simulink model "SecRwRtStFwdBkwdSpdCtrl"  (R2018b)
settings: Solver=FixedStepDiscrete  StartTime=0.0  StopTime=10.0  FixedStep=0.01  RelTol=1e-3
libraries: simulink x12
settings Model: Creator=sn2xws  LastModifiedBy=sn2xws
settings Model: ModifiedHistory=|
  | V2.4.0 Bug 655803  根据<REQ_MSM_697>修改调速
  | 2024.2.22
  | V2.5.0 Bug 732451增加模式15，18长滑轨调速
  | 2024.8.26 V3.0.0 557无长滑轨调速需求，发送默认值0
settings DataIOCC: SaveFormat=StructureWithTime
settings OptimizationCC: DefaultParameterBehavior=Inlined  EnhancedBackFolding=on  PassReuseOutputArgsAs=Individual arguments  ZeroExternalMemoryAtStartup=off  ZeroInternalMemoryAtStartup=off  OptimizeBlockOrder=speed  DifferentSizesBufferReuse=on  OptimizationCustomize=off
settings DebuggingCC: ParameterTunabilityLossMsg=error
settings ModelReferenceCC: ModelReferenceNumInstancesAllowed=Single
settings SFSimCC: MATLABDynamicMemAlloc=off
settings RTWCC: SystemTargetFile=autosar.tlc  GenCodeOnly=on  TemplateMakefile=ert_default_tmf  Description=AUTOSAR  GenerateReport=on  IncludeHyperlinkInReport=on  LaunchReport=on  GenerateTraceInfo=on  GenerateTraceReport=on  GenerateTraceReportSl=on  GenerateTraceReportSf=on  GenerateTraceReportEml=on  GenerateCodeMetricsReport=on
settings CodeAppCC: ForceParamTrailComments=on  IgnoreCustomStorageClasses=off  OperatorAnnotations=on  SimulinkDataObjDesc=on  SFDataObjDesc=on  InsertBlockDesc=on
settings STFCustomTargetCC: TargetLangStandard=C99 (ISO)  MultiwordLength=256  ParMdlRefBuildCompliant=on  CompOptLevelCompliant=on  IncludeMdlTerminateFcn=off  CombineOutputUpdateFcns=on  SuppressErrorStatus=on  ERTCustomFileBanners=on  SupportNonFinite=off  SupportComplex=off  SupportContinuousTime=off  SupportNonInlinedSFcns=off  RemoveResetFunc=on  MATLABClassNameForMDSCustomization=Simulink.SoftwareTarget.ERTCustomization  AutosarCompliant=on  UseToolchainInfoCompliant=on  LookupTableObjectStructAxisOrder=2,1,3,4,...  LUTObjectStructOrderEvenSpacing=Size,Table,Breakpoints  SystemTargetFile=autosar.tlc
settings ERTTargetCC: TargetLangStandard=C99 (ISO)  ConcurrentExecutionCompliant=off  IncludeMdlTerminateFcn=off  SuppressErrorStatus=on  SupportNonFinite=off  SupportComplex=off  ModelStepFunctionPrototypeControlCompliant=off  CPPClassGenCompliant=off  AutosarCompliant=on  LookupTableObjectStructAxisOrder=2,1,3,4,...  LUTObjectStructOrderEvenSpacing=Size,Table,Breakpoints  InlinedParameterPlacement=NonHierarchical  ERTCustomFileTemplate=example_file_process.tlc  ERTFilePackagingFormat=Compact

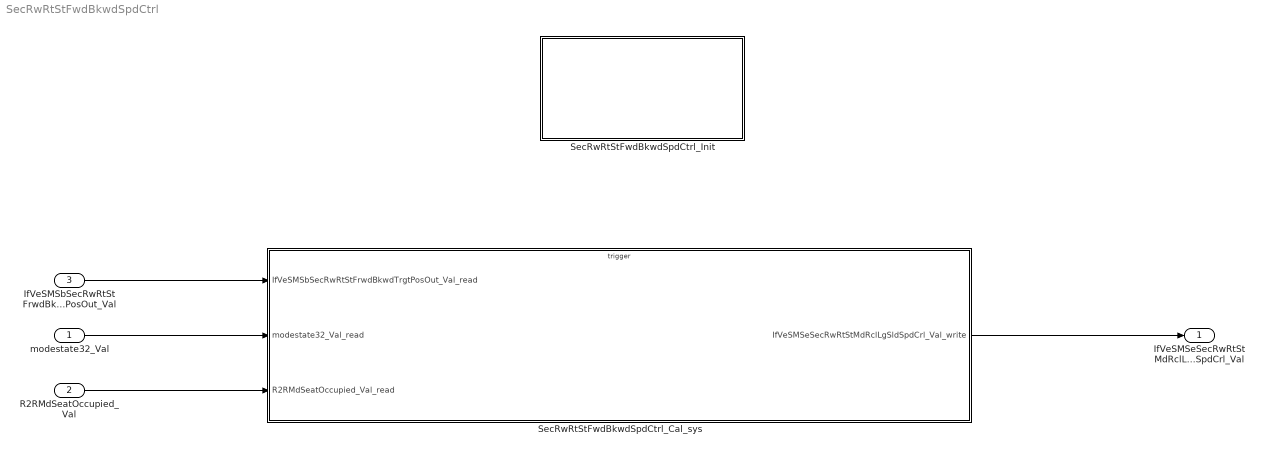
== system SecRwRtStFwdBkwdSpdCtrl ==
  modestate32_Val : Inport  OutDataTypeStr=uint32  PortDimensions=1
  R2RMdSeatOccupied_Val : Inport  Port=2  OutDataTypeStr=boolean  PortDimensions=1
  IfVeSMSbSecRwRtStFrwdBkwdTrgtPosOut_Val : Inport  Port=3  OutDataTypeStr=boolean  PortDimensions=1
  SecRwRtStFwdBkwdSpdCtrl_Cal_sys : Subsystem
  SecRwRtStFwdBkwdSpdCtrl_Init : Subsystem
  IfVeSMSeSecRwRtStMdRclLgSldSpdCrl_Val : Outport  OutDataTypeStr=uint8  PortDimensions=1
  wires:
  modestate32_Val/1 -> SecRwRtStFwdBkwdSpdCtrl_Cal_sys/2(modestate32_Val_read)
  R2RMdSeatOccupied_Val/1 -> SecRwRtStFwdBkwdSpdCtrl_Cal_sys/3(R2RMdSeatOccupied_Val_read)
  IfVeSMSbSecRwRtStFrwdBkwdTrgtPosOut_Val/1 -> SecRwRtStFwdBkwdSpdCtrl_Cal_sys/1(IfVeSMSbSecRwRtStFrwdBkwdTrgtPosOut_Val_read)
  SecRwRtStFwdBkwdSpdCtrl_Cal_sys/1(IfVeSMSeSecRwRtStMdRclLgSldSpdCrl_Val_write) -> IfVeSMSeSecRwRtStMdRclLgSldSpdCrl_Val/1

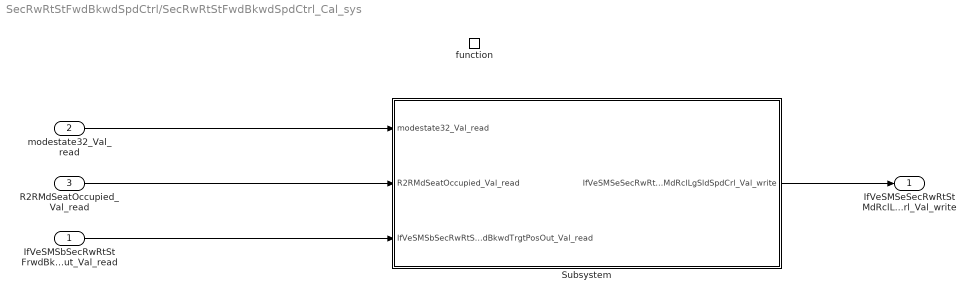
== system SecRwRtStFwdBkwdSpdCtrl/SecRwRtStFwdBkwdSpdCtrl_Cal_sys ==
  IfVeSMSbSecRwRtStFrwdBkwdTrgtPosOut_Val_read : Inport
  modestate32_Val_read : Inport  Port=2
  R2RMdSeatOccupied_Val_read : Inport  Port=3
  function : TriggerPort  TriggerType=function-call  IsSimulinkFunction=on  FunctionName=SecRwRtStFwdBkwdSpdCtrl_Cal  VariantControl=(inherit)
  Subsystem : Subsystem
  IfVeSMSeSecRwRtStMdRclLgSldSpdCrl_Val_write : Outport
      settings: EnsureOutportIsVirtual=on
  wires:
  Subsystem/1(IfVeSMSeSecRwRtStMdRclLgSldSpdCrl_Val_write) -> IfVeSMSeSecRwRtStMdRclLgSldSpdCrl_Val_write/1
  modestate32_Val_read/1 -> Subsystem/1(modestate32_Val_read)
  R2RMdSeatOccupied_Val_read/1 -> Subsystem/2(R2RMdSeatOccupied_Val_read)
  IfVeSMSbSecRwRtStFrwdBkwdTrgtPosOut_Val_read/1 -> Subsystem/3(IfVeSMSbSecRwRtStFrwdBkwdTrgtPosOut_Val_read)

== system SecRwRtStFwdBkwdSpdCtrl/SecRwRtStFwdBkwdSpdCtrl_Init ==
  Event Listener : EventListener  EventName=reset

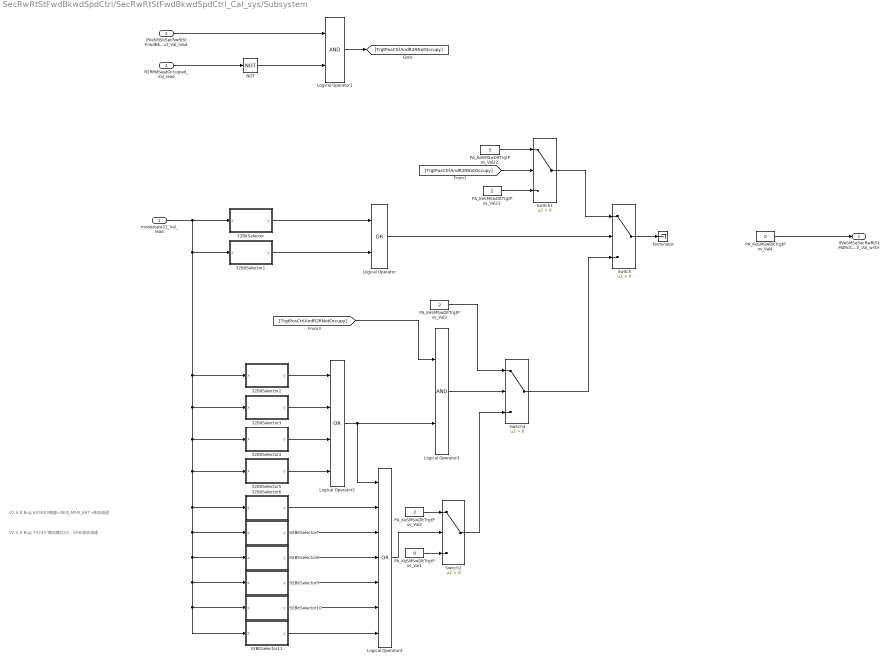
== system SecRwRtStFwdBkwdSpdCtrl/SecRwRtStFwdBkwdSpdCtrl_Cal_sys/Subsystem ==
  note: V2.5.0 Bug 732451增加模式15，18长滑轨调速
  note: V2.4.0 Bug 655803 根据<REQ_MSM_697>修改调速
  modestate32_Val_read : Inport
  R2RMdSeatOccupied_Val_read : Inport  Port=2
  IfVeSMSbSecRwRtStFrwdBkwdTrgtPosOut_Val_read : Inport  Port=3
  32BitSelector : Subsystem  mask(32 Bit Selector){BitNum=0}
      mask prompts: BitNum "Select Bit Number"
      mask help: Allows selection of a particular bit (0-31) out of a packed word up to 32 bits long. Output will be true if the bit number selected via the mask parameter is equal to one.
      mask TypeOptions BitNum: 0 | 1 | 2 | 3 | 4 | 5 | 6 | 7 | 8 | 9 | 10 | 11 | 12 | 13 | 14 | 15 | 16 | 17 | 18 | 19 | 20 | 21 | 22 | 23 | 24 | 25 | 26 | 27 | 28 | 29 | 30 | 31
      mask Display:
      | text(0.5, 0.8,'BIT','horizontalAlignment','center')
      | text(0.5, 0.5,'SELECTOR','horizontalAlignment','center')
      | text(0.5, 0.2,['-- Bit ',char(get_param(gcb,'BitNum')),' --'],'horizontalAlignment','center')
  32BitSelector1 : Subsystem  mask(32 Bit Selector){BitNum=3}
      mask prompts: BitNum "Select Bit Number"
      mask help: Allows selection of a particular bit (0-31) out of a packed word up to 32 bits long. Output will be true if the bit number selected via the mask parameter is equal to one.
      mask TypeOptions BitNum: 0 | 1 | 2 | 3 | 4 | 5 | 6 | 7 | 8 | 9 | 10 | 11 | 12 | 13 | 14 | 15 | 16 | 17 | 18 | 19 | 20 | 21 | 22 | 23 | 24 | 25 | 26 | 27 | 28 | 29 | 30 | 31
      mask Display:
      | text(0.5, 0.8,'BIT','horizontalAlignment','center')
      | text(0.5, 0.5,'SELECTOR','horizontalAlignment','center')
      | text(0.5, 0.2,['-- Bit ',char(get_param(gcb,'BitNum')),' --'],'horizontalAlignment','center')
  32BitSelector10 : Subsystem  mask(32 Bit Selector){BitNum=14}
      mask prompts: BitNum "Select Bit Number"
      mask help: Allows selection of a particular bit (0-31) out of a packed word up to 32 bits long. Output will be true if the bit number selected via the mask parameter is equal to one.
      mask TypeOptions BitNum: 0 | 1 | 2 | 3 | 4 | 5 | 6 | 7 | 8 | 9 | 10 | 11 | 12 | 13 | 14 | 15 | 16 | 17 | 18 | 19 | 20 | 21 | 22 | 23 | 24 | 25 | 26 | 27 | 28 | 29 | 30 | 31
      mask Display:
      | text(0.5, 0.8,'BIT','horizontalAlignment','center')
      | text(0.5, 0.5,'SELECTOR','horizontalAlignment','center')
      | text(0.5, 0.2,['-- Bit ',char(get_param(gcb,'BitNum')),' --'],'horizontalAlignment','center')
  32BitSelector11 : Subsystem  mask(32 Bit Selector){BitNum=17}
      mask prompts: BitNum "Select Bit Number"
      mask help: Allows selection of a particular bit (0-31) out of a packed word up to 32 bits long. Output will be true if the bit number selected via the mask parameter is equal to one.
      mask TypeOptions BitNum: 0 | 1 | 2 | 3 | 4 | 5 | 6 | 7 | 8 | 9 | 10 | 11 | 12 | 13 | 14 | 15 | 16 | 17 | 18 | 19 | 20 | 21 | 22 | 23 | 24 | 25 | 26 | 27 | 28 | 29 | 30 | 31
      mask Display:
      | text(0.5, 0.8,'BIT','horizontalAlignment','center')
      | text(0.5, 0.5,'SELECTOR','horizontalAlignment','center')
      | text(0.5, 0.2,['-- Bit ',char(get_param(gcb,'BitNum')),' --'],'horizontalAlignment','center')
  32BitSelector2 : Subsystem  mask(32 Bit Selector){BitNum=11}
      mask prompts: BitNum "Select Bit Number"
      mask help: Allows selection of a particular bit (0-31) out of a packed word up to 32 bits long. Output will be true if the bit number selected via the mask parameter is equal to one.
      mask TypeOptions BitNum: 0 | 1 | 2 | 3 | 4 | 5 | 6 | 7 | 8 | 9 | 10 | 11 | 12 | 13 | 14 | 15 | 16 | 17 | 18 | 19 | 20 | 21 | 22 | 23 | 24 | 25 | 26 | 27 | 28 | 29 | 30 | 31
      mask Display:
      | text(0.5, 0.8,'BIT','horizontalAlignment','center')
      | text(0.5, 0.5,'SELECTOR','horizontalAlignment','center')
      | text(0.5, 0.2,['-- Bit ',char(get_param(gcb,'BitNum')),' --'],'horizontalAlignment','center')
  32BitSelector3 : Subsystem  mask(32 Bit Selector){BitNum=19}
      mask prompts: BitNum "Select Bit Number"
      mask help: Allows selection of a particular bit (0-31) out of a packed word up to 32 bits long. Output will be true if the bit number selected via the mask parameter is equal to one.
      mask TypeOptions BitNum: 0 | 1 | 2 | 3 | 4 | 5 | 6 | 7 | 8 | 9 | 10 | 11 | 12 | 13 | 14 | 15 | 16 | 17 | 18 | 19 | 20 | 21 | 22 | 23 | 24 | 25 | 26 | 27 | 28 | 29 | 30 | 31
      mask Display:
      | text(0.5, 0.8,'BIT','horizontalAlignment','center')
      | text(0.5, 0.5,'SELECTOR','horizontalAlignment','center')
      | text(0.5, 0.2,['-- Bit ',char(get_param(gcb,'BitNum')),' --'],'horizontalAlignment','center')
  32BitSelector4 : Subsystem  mask(32 Bit Selector){BitNum=5}
      mask prompts: BitNum "Select Bit Number"
      mask help: Allows selection of a particular bit (0-31) out of a packed word up to 32 bits long. Output will be true if the bit number selected via the mask parameter is equal to one.
      mask TypeOptions BitNum: 0 | 1 | 2 | 3 | 4 | 5 | 6 | 7 | 8 | 9 | 10 | 11 | 12 | 13 | 14 | 15 | 16 | 17 | 18 | 19 | 20 | 21 | 22 | 23 | 24 | 25 | 26 | 27 | 28 | 29 | 30 | 31
      mask Display:
      | text(0.5, 0.8,'BIT','horizontalAlignment','center')
      | text(0.5, 0.5,'SELECTOR','horizontalAlignment','center')
      | text(0.5, 0.2,['-- Bit ',char(get_param(gcb,'BitNum')),' --'],'horizontalAlignment','center')
  32BitSelector5 : Subsystem  mask(32 Bit Selector){BitNum=6}
      mask prompts: BitNum "Select Bit Number"
      mask help: Allows selection of a particular bit (0-31) out of a packed word up to 32 bits long. Output will be true if the bit number selected via the mask parameter is equal to one.
      mask TypeOptions BitNum: 0 | 1 | 2 | 3 | 4 | 5 | 6 | 7 | 8 | 9 | 10 | 11 | 12 | 13 | 14 | 15 | 16 | 17 | 18 | 19 | 20 | 21 | 22 | 23 | 24 | 25 | 26 | 27 | 28 | 29 | 30 | 31
      mask Display:
      | text(0.5, 0.8,'BIT','horizontalAlignment','center')
      | text(0.5, 0.5,'SELECTOR','horizontalAlignment','center')
      | text(0.5, 0.2,['-- Bit ',char(get_param(gcb,'BitNum')),' --'],'horizontalAlignment','center')
  32BitSelector6 : Subsystem  mask(32 Bit Selector){BitNum=22}
      mask prompts: BitNum "Select Bit Number"
      mask help: Allows selection of a particular bit (0-31) out of a packed word up to 32 bits long. Output will be true if the bit number selected via the mask parameter is equal to one.
      mask TypeOptions BitNum: 0 | 1 | 2 | 3 | 4 | 5 | 6 | 7 | 8 | 9 | 10 | 11 | 12 | 13 | 14 | 15 | 16 | 17 | 18 | 19 | 20 | 21 | 22 | 23 | 24 | 25 | 26 | 27 | 28 | 29 | 30 | 31
      mask Display:
      | text(0.5, 0.8,'BIT','horizontalAlignment','center')
      | text(0.5, 0.5,'SELECTOR','horizontalAlignment','center')
      | text(0.5, 0.2,['-- Bit ',char(get_param(gcb,'BitNum')),' --'],'horizontalAlignment','center')
  32BitSelector7 : Subsystem  mask(32 Bit Selector){BitNum=23}
      mask prompts: BitNum "Select Bit Number"
      mask help: Allows selection of a particular bit (0-31) out of a packed word up to 32 bits long. Output will be true if the bit number selected via the mask parameter is equal to one.
      mask TypeOptions BitNum: 0 | 1 | 2 | 3 | 4 | 5 | 6 | 7 | 8 | 9 | 10 | 11 | 12 | 13 | 14 | 15 | 16 | 17 | 18 | 19 | 20 | 21 | 22 | 23 | 24 | 25 | 26 | 27 | 28 | 29 | 30 | 31
      mask Display:
      | text(0.5, 0.8,'BIT','horizontalAlignment','center')
      | text(0.5, 0.5,'SELECTOR','horizontalAlignment','center')
      | text(0.5, 0.2,['-- Bit ',char(get_param(gcb,'BitNum')),' --'],'horizontalAlignment','center')
  32BitSelector8 : Subsystem  mask(32 Bit Selector){BitNum=24}
      mask prompts: BitNum "Select Bit Number"
      mask help: Allows selection of a particular bit (0-31) out of a packed word up to 32 bits long. Output will be true if the bit number selected via the mask parameter is equal to one.
      mask TypeOptions BitNum: 0 | 1 | 2 | 3 | 4 | 5 | 6 | 7 | 8 | 9 | 10 | 11 | 12 | 13 | 14 | 15 | 16 | 17 | 18 | 19 | 20 | 21 | 22 | 23 | 24 | 25 | 26 | 27 | 28 | 29 | 30 | 31
      mask Display:
      | text(0.5, 0.8,'BIT','horizontalAlignment','center')
      | text(0.5, 0.5,'SELECTOR','horizontalAlignment','center')
      | text(0.5, 0.2,['-- Bit ',char(get_param(gcb,'BitNum')),' --'],'horizontalAlignment','center')
  32BitSelector9 : Subsystem  mask(32 Bit Selector){BitNum=25}
      mask prompts: BitNum "Select Bit Number"
      mask help: Allows selection of a particular bit (0-31) out of a packed word up to 32 bits long. Output will be true if the bit number selected via the mask parameter is equal to one.
      mask TypeOptions BitNum: 0 | 1 | 2 | 3 | 4 | 5 | 6 | 7 | 8 | 9 | 10 | 11 | 12 | 13 | 14 | 15 | 16 | 17 | 18 | 19 | 20 | 21 | 22 | 23 | 24 | 25 | 26 | 27 | 28 | 29 | 30 | 31
      mask Display:
      | text(0.5, 0.8,'BIT','horizontalAlignment','center')
      | text(0.5, 0.5,'SELECTOR','horizontalAlignment','center')
      | text(0.5, 0.2,['-- Bit ',char(get_param(gcb,'BitNum')),' --'],'horizontalAlignment','center')
  Logical Operator : Logic  Operator=OR  AllPortsSameDT=off  OutDataTypeStr=boolean
  Logical Operator1 : Logic  AllPortsSameDT=off  OutDataTypeStr=boolean
  Logical Operator2 : Logic  Operator=OR  Inputs=4  AllPortsSameDT=off  OutDataTypeStr=boolean
  Logical Operator3 : Logic  AllPortsSameDT=off  OutDataTypeStr=boolean
  Logical Operator4 : Logic  Operator=OR  Inputs=7  AllPortsSameDT=off  OutDataTypeStr=boolean
  NOT : Logic  Operator=NOT  AllPortsSameDT=off  OutDataTypeStr=boolean
  PA_KeSMSwDltTrgtPos_Val1 : Constant  Value=0  OutDataTypeStr=uint8
  PA_KeSMSwDltTrgtPos_Val2 : Constant  Value=2  OutDataTypeStr=uint8
  PA_KeSMSwDltTrgtPos_Val22 : Constant  Value=3  OutDataTypeStr=uint8
  PA_KeSMSwDltTrgtPos_Val23 : Constant  Value=2  OutDataTypeStr=uint8
  PA_KeSMSwDltTrgtPos_Val3 : Constant  Value=2  OutDataTypeStr=uint8
  PA_KeSMSwDltTrgtPos_Val4 : Constant  Value=0  OutDataTypeStr=uint8
  Switch{,1..2,4} (4 alike) : Switch  Criteria=u2 > Threshold
  Terminator : Terminator
  IfVeSMSeSecRwRtStMdRclLgSldSpdCrl_Val_write : Outport
      settings: EnsureOutportIsVirtual=on
  wires:
  IfVeSMSbSecRwRtStFrwdBkwdTrgtPosOut_Val_read/1 -> Logical Operator1/1
  NOT/1 -> Logical Operator1/2
  R2RMdSeatOccupied_Val_read/1 -> NOT/1
  Logical Operator1/1 -> [TrgtPosCtrlAndR2RNotOccupy]
  Logical Operator/1 -> Switch/2
  32BitSelector/1(y) -> Logical Operator/1
  32BitSelector1/1(y) -> Logical Operator/2
  Switch4/1 -> Switch/3
  PA_KeSMSwDltTrgtPos_Val22/1 -> Switch1/1
  Switch1/1 -> Switch/1
  [TrgtPosCtrlAndR2RNotOccupy] -> Switch1/2
  PA_KeSMSwDltTrgtPos_Val23/1 -> Switch1/3
  32BitSelector3/1(y) -> Logical Operator2/2
  32BitSelector5/1(y) -> Logical Operator2/4
  Logical Operator2/1 -> Logical Operator4/1, Logical Operator3/2
  32BitSelector2/1(y) -> Logical Operator2/1
  32BitSelector4/1(y) -> Logical Operator2/3
  [TrgtPosCtrlAndR2RNotOccupy] -> Logical Operator3/1
  modestate32_Val_read/1 -> 32BitSelector4/1(x), 32BitSelector11/1(x), 32BitSelector10/1(x), 32BitSelector9/1(x), 32BitSelector8/1(x), 32BitSelector7/1(x), 32BitSelector6/1(x), 32BitSelector5/1(x), 32BitSelector3/1(x), 32BitSelector2/1(x), 32BitSelector1/1(x), 32BitSelector/1(x)
  PA_KeSMSwDltTrgtPos_Val3/1 -> Switch4/1
  Logical Operator3/1 -> Switch4/2
  Switch2/1 -> Switch4/3
  Logical Operator4/1 -> Switch2/2
  PA_KeSMSwDltTrgtPos_Val1/1 -> Switch2/3
  PA_KeSMSwDltTrgtPos_Val2/1 -> Switch2/1
  32BitSelector6/1(y) -> Logical Operator4/2
  32BitSelector7/1(y) -> Logical Operator4/3
  32BitSelector8/1(y) -> Logical Operator4/4
  32BitSelector9/1(y) -> Logical Operator4/5
  32BitSelector11/1(y) -> Logical Operator4/7
  32BitSelector10/1(y) -> Logical Operator4/6
  PA_KeSMSwDltTrgtPos_Val4/1 -> IfVeSMSeSecRwRtStMdRclLgSldSpdCrl_Val_write/1
  Switch/1 -> Terminator/1

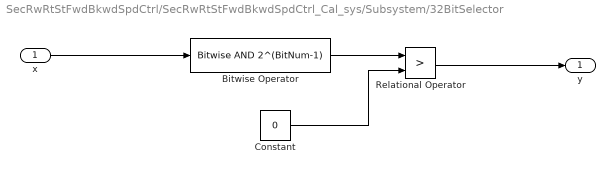
== system SecRwRtStFwdBkwdSpdCtrl/SecRwRtStFwdBkwdSpdCtrl_Cal_sys/Subsystem/32BitSelector ==
  x : Inport
  Bitwise Operator : simulink/Logic and Bit Operations/Bitwise Operator  logicop=AND  UseBitMask=on  BitMask=2^(BitNum-1)  BitMaskRealWorld=Stored Integer
  Constant : Constant  Value=0  OutDataTypeStr=uint32
  Relational Operator : RelationalOperator  Operator=>  OutDataTypeStr=boolean  RndMeth=Simplest
  y : Outport
  wires:
  Relational Operator/1 -> y/1
  Constant/1 -> Relational Operator/2
  x/1 -> Bitwise Operator/1
  Bitwise Operator/1 -> Relational Operator/1

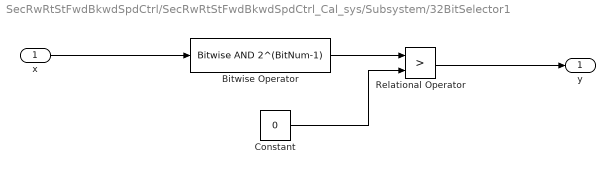
== system SecRwRtStFwdBkwdSpdCtrl/SecRwRtStFwdBkwdSpdCtrl_Cal_sys/Subsystem/32BitSelector1 ==
  x : Inport
  Bitwise Operator : simulink/Logic and Bit Operations/Bitwise Operator  logicop=AND  UseBitMask=on  BitMask=2^(BitNum-1)  BitMaskRealWorld=Stored Integer
  Constant : Constant  Value=0  OutDataTypeStr=uint32
  Relational Operator : RelationalOperator  Operator=>  OutDataTypeStr=boolean  RndMeth=Simplest
  y : Outport
  wires:
  Bitwise Operator/1 -> Relational Operator/1
  x/1 -> Bitwise Operator/1
  Constant/1 -> Relational Operator/2
  Relational Operator/1 -> y/1

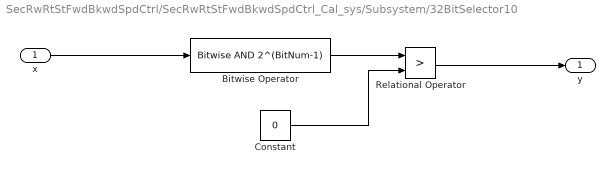
== system SecRwRtStFwdBkwdSpdCtrl/SecRwRtStFwdBkwdSpdCtrl_Cal_sys/Subsystem/32BitSelector10 ==
  x : Inport
  Bitwise Operator : simulink/Logic and Bit Operations/Bitwise Operator  logicop=AND  UseBitMask=on  BitMask=2^(BitNum-1)  BitMaskRealWorld=Stored Integer
  Constant : Constant  Value=0  OutDataTypeStr=uint32
  Relational Operator : RelationalOperator  Operator=>  OutDataTypeStr=boolean  RndMeth=Simplest
  y : Outport
  wires:
  Relational Operator/1 -> y/1
  Constant/1 -> Relational Operator/2
  x/1 -> Bitwise Operator/1
  Bitwise Operator/1 -> Relational Operator/1

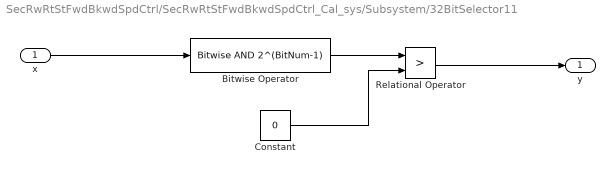
== system SecRwRtStFwdBkwdSpdCtrl/SecRwRtStFwdBkwdSpdCtrl_Cal_sys/Subsystem/32BitSelector11 ==
  x : Inport
  Bitwise Operator : simulink/Logic and Bit Operations/Bitwise Operator  logicop=AND  UseBitMask=on  BitMask=2^(BitNum-1)  BitMaskRealWorld=Stored Integer
  Constant : Constant  Value=0  OutDataTypeStr=uint32
  Relational Operator : RelationalOperator  Operator=>  OutDataTypeStr=boolean  RndMeth=Simplest
  y : Outport
  wires:
  Bitwise Operator/1 -> Relational Operator/1
  x/1 -> Bitwise Operator/1
  Constant/1 -> Relational Operator/2
  Relational Operator/1 -> y/1

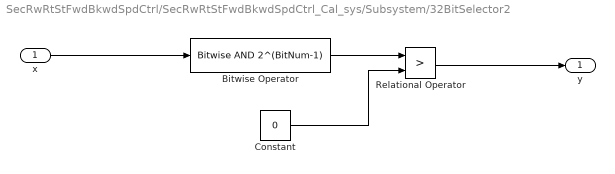
== system SecRwRtStFwdBkwdSpdCtrl/SecRwRtStFwdBkwdSpdCtrl_Cal_sys/Subsystem/32BitSelector2 ==
  x : Inport
  Bitwise Operator : simulink/Logic and Bit Operations/Bitwise Operator  logicop=AND  UseBitMask=on  BitMask=2^(BitNum-1)  BitMaskRealWorld=Stored Integer
  Constant : Constant  Value=0  OutDataTypeStr=uint32
  Relational Operator : RelationalOperator  Operator=>  OutDataTypeStr=boolean  RndMeth=Simplest
  y : Outport
  wires:
  Relational Operator/1 -> y/1
  Constant/1 -> Relational Operator/2
  x/1 -> Bitwise Operator/1
  Bitwise Operator/1 -> Relational Operator/1

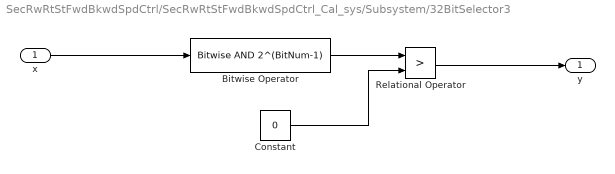
== system SecRwRtStFwdBkwdSpdCtrl/SecRwRtStFwdBkwdSpdCtrl_Cal_sys/Subsystem/32BitSelector3 ==
  x : Inport
  Bitwise Operator : simulink/Logic and Bit Operations/Bitwise Operator  logicop=AND  UseBitMask=on  BitMask=2^(BitNum-1)  BitMaskRealWorld=Stored Integer
  Constant : Constant  Value=0  OutDataTypeStr=uint32
  Relational Operator : RelationalOperator  Operator=>  OutDataTypeStr=boolean  RndMeth=Simplest
  y : Outport
  wires:
  Bitwise Operator/1 -> Relational Operator/1
  x/1 -> Bitwise Operator/1
  Constant/1 -> Relational Operator/2
  Relational Operator/1 -> y/1

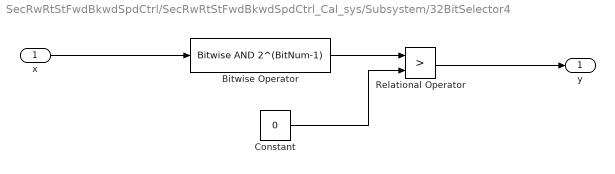
== system SecRwRtStFwdBkwdSpdCtrl/SecRwRtStFwdBkwdSpdCtrl_Cal_sys/Subsystem/32BitSelector4 ==
  x : Inport
  Bitwise Operator : simulink/Logic and Bit Operations/Bitwise Operator  logicop=AND  UseBitMask=on  BitMask=2^(BitNum-1)  BitMaskRealWorld=Stored Integer
  Constant : Constant  Value=0  OutDataTypeStr=uint32
  Relational Operator : RelationalOperator  Operator=>  OutDataTypeStr=boolean  RndMeth=Simplest
  y : Outport
  wires:
  Relational Operator/1 -> y/1
  Constant/1 -> Relational Operator/2
  x/1 -> Bitwise Operator/1
  Bitwise Operator/1 -> Relational Operator/1

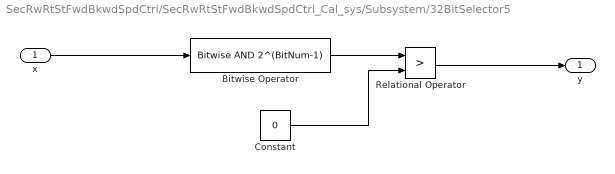
== system SecRwRtStFwdBkwdSpdCtrl/SecRwRtStFwdBkwdSpdCtrl_Cal_sys/Subsystem/32BitSelector5 ==
  x : Inport
  Bitwise Operator : simulink/Logic and Bit Operations/Bitwise Operator  logicop=AND  UseBitMask=on  BitMask=2^(BitNum-1)  BitMaskRealWorld=Stored Integer
  Constant : Constant  Value=0  OutDataTypeStr=uint32
  Relational Operator : RelationalOperator  Operator=>  OutDataTypeStr=boolean  RndMeth=Simplest
  y : Outport
  wires:
  Bitwise Operator/1 -> Relational Operator/1
  x/1 -> Bitwise Operator/1
  Constant/1 -> Relational Operator/2
  Relational Operator/1 -> y/1

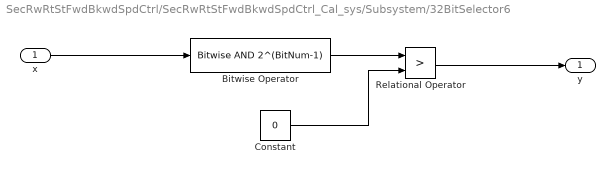
== system SecRwRtStFwdBkwdSpdCtrl/SecRwRtStFwdBkwdSpdCtrl_Cal_sys/Subsystem/32BitSelector6 ==
  x : Inport
  Bitwise Operator : simulink/Logic and Bit Operations/Bitwise Operator  logicop=AND  UseBitMask=on  BitMask=2^(BitNum-1)  BitMaskRealWorld=Stored Integer
  Constant : Constant  Value=0  OutDataTypeStr=uint32
  Relational Operator : RelationalOperator  Operator=>  OutDataTypeStr=boolean  RndMeth=Simplest
  y : Outport
  wires:
  Relational Operator/1 -> y/1
  Constant/1 -> Relational Operator/2
  x/1 -> Bitwise Operator/1
  Bitwise Operator/1 -> Relational Operator/1

== system SecRwRtStFwdBkwdSpdCtrl/SecRwRtStFwdBkwdSpdCtrl_Cal_sys/Subsystem/32BitSelector7 ==
  x : Inport
  Bitwise Operator : simulink/Logic and Bit Operations/Bitwise Operator  logicop=AND  UseBitMask=on  BitMask=2^(BitNum-1)  BitMaskRealWorld=Stored Integer
  Constant : Constant  Value=0  OutDataTypeStr=uint32
  Relational Operator : RelationalOperator  Operator=>  OutDataTypeStr=boolean  RndMeth=Simplest
  y : Outport
  wires:
  Bitwise Operator/1 -> Relational Operator/1
  x/1 -> Bitwise Operator/1
  Constant/1 -> Relational Operator/2
  Relational Operator/1 -> y/1

== system SecRwRtStFwdBkwdSpdCtrl/SecRwRtStFwdBkwdSpdCtrl_Cal_sys/Subsystem/32BitSelector8 ==
  x : Inport
  Bitwise Operator : simulink/Logic and Bit Operations/Bitwise Operator  logicop=AND  UseBitMask=on  BitMask=2^(BitNum-1)  BitMaskRealWorld=Stored Integer
  Constant : Constant  Value=0  OutDataTypeStr=uint32
  Relational Operator : RelationalOperator  Operator=>  OutDataTypeStr=boolean  RndMeth=Simplest
  y : Outport
  wires:
  Relational Operator/1 -> y/1
  Constant/1 -> Relational Operator/2
  x/1 -> Bitwise Operator/1
  Bitwise Operator/1 -> Relational Operator/1

== system SecRwRtStFwdBkwdSpdCtrl/SecRwRtStFwdBkwdSpdCtrl_Cal_sys/Subsystem/32BitSelector9 ==
  x : Inport
  Bitwise Operator : simulink/Logic and Bit Operations/Bitwise Operator  logicop=AND  UseBitMask=on  BitMask=2^(BitNum-1)  BitMaskRealWorld=Stored Integer
  Constant : Constant  Value=0  OutDataTypeStr=uint32
  Relational Operator : RelationalOperator  Operator=>  OutDataTypeStr=boolean  RndMeth=Simplest
  y : Outport
  wires:
  Bitwise Operator/1 -> Relational Operator/1
  x/1 -> Bitwise Operator/1
  Constant/1 -> Relational Operator/2
  Relational Operator/1 -> y/1
